simulink model "gravity_operational"  (R2023a)
settings: Solver=VariableStepAuto  StartTime=0.0  StopTime=10.0  RelTol=1e-3
undefined symbols (not defined in the file): dqi, Kd, Kp, qi, robot, xd
settings Model: Creator=franc  LastModifiedBy=franc

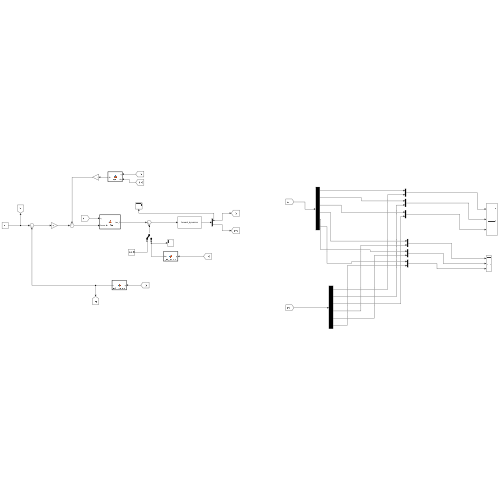
[thumbnail: Simulink's stored preview of the top-level diagram]
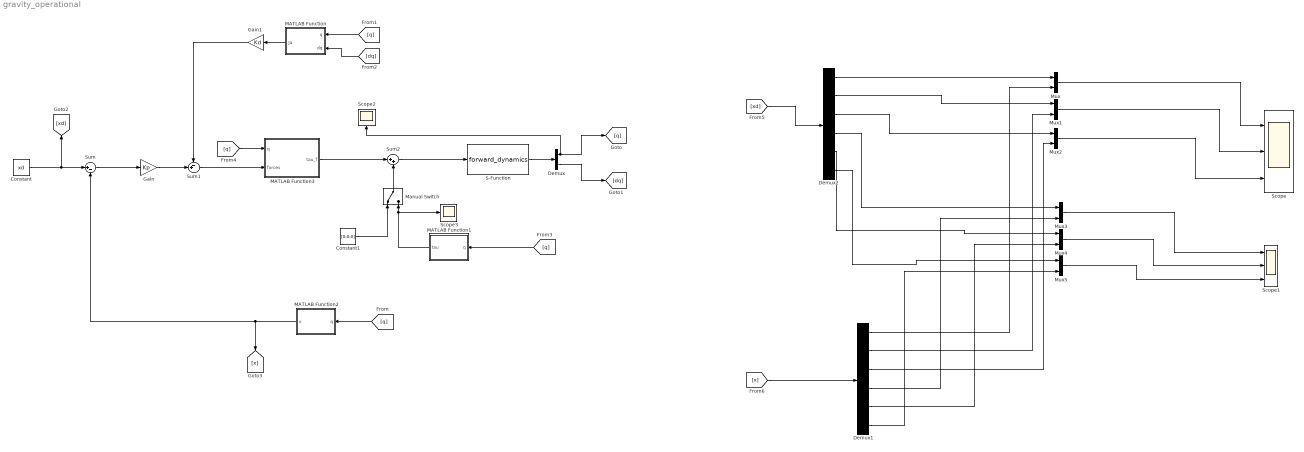
== system gravity_operational ==
  Constant : Constant  Value=xd
  Constant1 : Constant  Value=[0;0;0]
  Demux : Demux  Outputs=2
  Demux1 : Demux  Outputs=6
  Demux2 : Demux  Outputs=6
  Gain : Gain  Gain=Kp
  Gain1 : Gain  Gain=Kd
  MATLAB Function : MATLAB Function  TreatAsAtomicUnit=on
  MATLAB Function1 : MATLAB Function  TreatAsAtomicUnit=on
  MATLAB Function2 : MATLAB Function  TreatAsAtomicUnit=on
  MATLAB Function3 : MATLAB Function  TreatAsAtomicUnit=on
  Manual Switch : ManualSwitch
  Mux{,1..5} (6 alike) : Mux  Inputs=2
  S-Function : S-Function  FunctionName=forward_dynamics  Parameters=robot,qi,dqi  SFunctionDeploymentMode=off  EnableBusSupport=off
  Scope : Scope  NumInputPorts=3
  Scope1 : Scope  NumInputPorts=3
  Scope2 : Scope
  Scope3 : Scope
  Sum : Sum  Inputs=|+-
  Sum1 : Sum  Inputs=-+|
  Sum2 : Sum  Inputs=|++
  wires:
  Constant/1 -> [xd], Sum/1
  Sum/1 -> Gain/1
  Gain/1 -> Sum1/2
  Gain1/1 -> Sum1/1
  Sum2/1 -> S-Function/1
  S-Function/1 -> Demux/1
  Demux/1 -> Scope2/1, [q]
  Demux/2 -> [dq]
  MATLAB Function2/1(x) -> [x], Sum/2
  [q] -> MATLAB Function2/1(q)
  [dq] -> MATLAB Function/2(dq)
  [q] -> MATLAB Function/1(q)
  MATLAB Function/1(Ja) -> Gain1/1
  [q] -> MATLAB Function1/1(q)
  Sum1/1 -> MATLAB Function3/2(forces)
  [q] -> MATLAB Function3/1(q)
  MATLAB Function3/1(tau_f) -> Sum2/1
  [x] -> Demux1/1
  [xd] -> Demux2/1
  Demux2/1 -> Mux/1
  Demux2/2 -> Mux1/1
  Demux2/3 -> Mux2/1
  Demux2/4 -> Mux3/1
  Demux2/5 -> Mux4/1
  Demux2/6 -> Mux5/1
  Demux1/1 -> Mux/2
  Demux1/2 -> Mux1/2
  Demux1/3 -> Mux2/2
  Demux1/4 -> Mux3/2
  Demux1/5 -> Mux4/2
  Demux1/6 -> Mux5/2
  Mux/1 -> Scope/1
  Mux1/1 -> Scope/2
  Mux2/1 -> Scope/3
  Mux3/1 -> Scope1/1
  Mux4/1 -> Scope1/2
  Mux5/1 -> Scope1/3
  Manual Switch/1 -> Sum2/2
  MATLAB Function1/1(tau) -> Manual Switch/2, Scope3/1
  Constant1/1 -> Manual Switch/1

== matlab function gravity_operational/MATLAB Function ==
  data: q input; Ja output; dq input
function Ja = fcn(q,dq)
Ja = zeros(6,1);
Ja = get_Ja_as_9(q(1),q(2),q(3))*dq;

== matlab function gravity_operational/MATLAB Function2 ==
  data: q input; x output
function x = get_cartesian(q)

x = get_k_as_9(q(1),q(2),q(3));

end

== matlab function gravity_operational/MATLAB Function3 ==
  data: q input; tau_f output; forces input
function tau_f = get_tau(q,forces)
    tau_f = zeros(3,1);
    tau_f = (get_Ja_as_9(q(1),q(2),q(3)))' * forces;

end

== matlab function gravity_operational/MATLAB Function1 ==
  data: q input; tau output
function tau = get_gravity(q)
    tau = zeros(3,1);
    tau = get_G_as_9(q(1),q(2),q(3));

end
